simulink model "qpsk_modulation_and_demodulation_1"  (R2024a)
settings: Solver=VariableStepAuto  StartTime=0.0  StopTime=inf  RelTol=1e-3
libraries: simulink x4, dspfdesign x3, dspsigops x3, commsync2 x2, commrflib2 x2, dspxfrm3 x1, commdigbbndpm3 x1, sdrrlib x1, commfilt2 x1, matrix_library x1
settings Model: SimulationMode=accelerator  Creator=digital  LastModifiedBy=opr

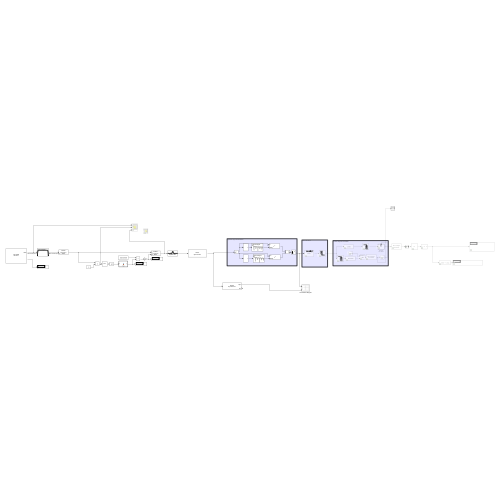
[thumbnail: Simulink's stored preview of the top-level diagram]
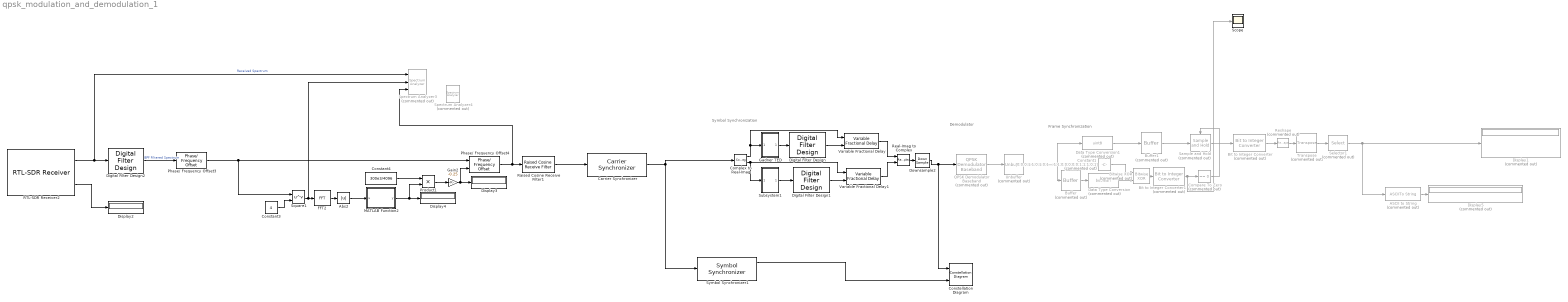
== system qpsk_modulation_and_demodulation_1 ==
  note: Frame Synchronization
  note: Demodulator
  note: Symbol Synchronization
  ASCII to String : ASCIIToString  Commented=on
  Abs2 : Abs  SaturateOnIntegerOverflow=off
  Bit to Integer Converter : simulink/Logic and Bit Operations/Bit to Integer Converter  Commented=on  nbits=8  bitOrder=MSB first  signedOutputValues=Unsigned  outDtype=Inherit via internal rule  outDtypeSigned=Inherit via internal rule
  Bit to Integer Converter1 : simulink/Logic and Bit Operations/Bit to Integer Converter  Commented=on  nbits=32  bitOrder=MSB first  signedOutputValues=Unsigned  outDtype=Inherit via internal rule  outDtypeSigned=Inherit via internal rule
  Bitwise XOR : simulink/Logic and Bit Operations/Bitwise Operator  Commented=on  logicop=XOR  UseBitMask=off  NumInputPorts=2  BitMask=bin2dec('11011001')  BitMaskRealWorld=Stored Integer
      settings: LibrarySourceBlock=|
      | simulink/Quick Insert/Logic and Bit
      | Operations/Bitwise XOR
  Buffer : Buffer  Commented=on  N=32  V=31  OutputFrames=off
  Buffer1 : Buffer  Commented=on  N=160  V=159  OutputFrames=off
  Carrier Synchronizer : commsync2/Carrier Synchronizer  Modulation=QPSK  ModulationPhaseOffset=Auto  CustomPhaseOffset=0  SamplesPerSymbol=2  DampingFactor=0.707  NormalizedLoopBandwidth=0.01  EstimatedPhaseErrorOutputPort=off  SimulateUsing=Code generation
  Compare To Zero : simulink/Logic and Bit Operations/Compare To Zero  Commented=on  relop===  OutDataTypeStr=boolean
  Complex to Real-Imag : ComplexToRealImag
  Constant1 : Constant  Commented=on  Value=[0;0;0;1;1;0;1;0;1;1;0;0;1;1;1;1;1;1;1;1;1;1;0;0;0;0;0;1;1;1;0;1]  VectorParams1D=off  OutDataTypeStr=boolean  SampleTime=1/10e6
  Constant3 : Constant  Value=4
  Constant4 : Constant  Value=300e3/4096
  Constellation Diagram : ConstellationDiagram  NumInputPorts=2  WindowPosition=[1.000000,49.000000,2048.000000,1080.000000,]  ScopeFrameLocation=window  ReferenceConstellation="{[0.7071+0.7071i          -0.7071+0.7071i          -0.7071-0.7071i            0.707-0.7071i][0.7071+0.7071i          -0.7071+0.7071i          -0.7071-0.7071i            0.707-0.7071i]}"  ShowLegend=on
  Data Type Conversion : DataTypeConversion  Commented=on  OutDataTypeStr=boolean  SaturateOnIntegerOverflow=off  RndMeth=Floor
  Data Type Conversion1 : DataTypeConversion  Commented=on  OutDataTypeStr=uint8  SaturateOnIntegerOverflow=off  RndMeth=Floor
  Digital Filter Design : dspfdesign/Digital Filter Design  mwdsp_browser_bugfix_var=off
  Digital Filter Design1 : dspfdesign/Digital Filter Design  mwdsp_browser_bugfix_var=off
  Digital Filter Design2 : dspfdesign/Digital Filter Design  mwdsp_browser_bugfix_var=off
  Display1 : Display  Commented=on
      settings: Format=hex (Stored Integer)
  Display2 : Display
  Display3 : Display
  Display4 : Display
  Display5 : Display  Commented=on
  Downsample2 : DownSample  RateOptions=Allow multirate processing  AllowArbitraryFixedInput=on
  FFT2 : dspxfrm3/FFT  FFTImplementation=Auto  CompMethod=Table lookup  TableOpt=NEW  TableOptActive=Speed  BitRevOrder=off  Normalize=off  InheritFFTLength=on  FFTLength=64  WrapInput=on  roundingMode=Ceiling  overflowMode=off  firstCoeffDataTypeStr=Inherit: Same word length as input  firstCoeffLastDataTypeStr=Inherit: Same word length as input  outputMin=[]  outputMax=[]
  Gadner TED : Subsystem
  Gain2 : Gain  Gain=-0.25
  MATLAB Function2 : MATLAB Function  TreatAsAtomicUnit=on
  Phase/ Frequency Offset3 : commrflib2/Phase// Frequency Offset  phaseOffset=0  freqPort=off  freqOffset=-(300e3)/8
  Phase/ Frequency Offset4 : commrflib2/Phase// Frequency Offset  phaseOffset=0  freqPort=on  freqOffset=500e6
  Product1 : Product
  QPSK Demodulator Baseband : commdigbbndpm3/QPSK Demodulator Baseband  Commented=on  OutType=Bit  DecType=Hard decision  VarSource=Dialog  Variance=1  Dec=Gray  Ph=pi/4  outDtype1=double  outDtype2=uint8  derotateFactorWordLen=16  derotateFactorDataTypeStr=Inherit: Same word length as input  derotateFactorLastDataTypeStr=Inherit: Same word length as input
  RTL-SDR Receiver2 : sdrrlib/RTL-SDR Receiver  IPAddress=0  CenterFrequencySource=Dialog  CenterFrequency=450e6 - (300e3)/4  GainSource=Dialog  Gain=10  ADCRate=300e3  FrequencyCorrection=0  LostSamplesOutputPort=on  LatencyOutputPort=off  OutputDataType=double  FrameLength=4096  EnableBurstMode=off  NumFramesInBurst=50  sobjType=sdrr.internal.SDRRTLReceiverSL  dataUDPPort=-1  ctrlUDPPort=-1  subDeviceList=nosubdev  sdrBlockType=SDRBlockTypeSLT.SDRRxBlock  requester=UNUSED_BY_SFCN  sdrExecutionMode=SDRExecutionModeSLT.ExecModeHW  BypassUserLogic=off  DecimatorSelect=DDC decimator  SourceSelect=RF data  SineAmplitude=16000  EnableInternalClock=off  BypassIQBalance=off  IFBandwidth=40e6  ADCRateSource=Dialog  IntermediateFrequency=0  DecimationFactorSource=Dialog  DecimationFactor=512  RFFrequencyIsTunable=logical(0)  SampleTime=(4096)/(300e3)  IFBandwidthSource=Dialog  SineFrequency=30000  BypassDCBlockingFilter=off  IntermediateFrequencySource=Dialog  IQBalanceCoefficients=64  SkipAllHardwareResetAndInitialization=off  EnableIQCalibrationTable=on  CacheIQCalibrationTable=off  EnableOffsetTuning=off  EnableRTLAGC=off  EnableTestMode=off  EnableTunerAGC=off  FrequencyCorrectionSource=Dialog  NumMLBuffers=128  NumUSBBuffers=16  RTLCrystalFrequency=28800000  TunerCrystalFrequency=28800000
  Raised Cosine Receive Filter1 : commfilt2/Raised Cosine Receive Filter  filtType=Square root  R=0.2  filtSpan=10  N=12  downFactor=6  downOffset=0  filterGain=1  InputProcessing=Columns as channels (frame based)  RateOptions=Allow multirate processing  framing=Mute  checkCoeff=off  variableName=rcRxFilt1  currentFiltSpan=10  D=5  inputOffset=0  sampMode=Mute  saveAsFlag=0  rateMode=Downsampling  checkGain=Normalized  launchFVT=on  roundingMode=Floor  overflowMode=off  coeffDataTypeStr=Inherit: Same word length as input  coeffMin=[]  coeffMax=[]  coeffLastDataTypeStr=Inherit: Same word length as input  accumDataTypeStr=Inherit: Same as product output  accumLastDataTypeStr=Inherit: Same as product output  outputDataTypeStr=Inherit: Same as accumulator  outputMin=[]  outputMax=[]  outputLastDataTypeStr=Inherit: Same as accumulator
  Real-Imag to Complex : RealImagToComplex
  Reshape : Reshape  Commented=on  OutputDimensionality=Row vector (2-D)  OutputDimensions=[1,]
  Sample and Hold : dspsigops/Sample and Hold  Commented=on  trig=Rising edge  initCond=0  latchinput=off
  Scope : Scope
  Selector1 : Selector  Commented=on  InputPortWidth=20  IndexOptions=Index vector (dialog)  Indices=[5:15]  OutputSizes=1
  Spectrum Analyzer3 : SpectrumAnalyzer  Commented=on  NumInputPorts=3  WindowPosition=[111.000000,294.000000,842.000000,726.000000,]  ScopeFrameLocation=window  YLimits=[-283.1209233885463,30.99910976663294]  ShowLegend=on  ExpandToolstrip=on  SelectedToolstripTab=spectrumAnalyzerToolstrip.measurementsTab
  Spectrum Analyzer4 : SpectrumAnalyzer  Commented=on  NumInputPorts=2  WindowPosition=[1367.000000,49.000000,680.000000,1072.000000,]  ScopeFrameLocation=window  YLimits=[-671.6431784277555,755.4983202728769]  ShowLegend=on  SelectedToolstripTab=spectrumAnalyzerToolstrip.measurementsTab
  Square1 : Math  Operator=pow
  Subsystem1 : Subsystem
  Symbol Synchronizer1 : commsync2/Symbol Synchronizer  Modulation=PAM/PSK/QAM  TimingErrorDetector=Gardner (non-data-aided)  SamplesPerSymbol=2  DampingFactor=1  NormalizedLoopBandwidth=0.01  DetectorGain=2.7  TimingErrorOutputPort=on  SimulateUsing=Interpreted execution
  Transpose : matrix_library/Transpose  Commented=on
  Unbuffer : Unbuffer  Commented=on
  Variable Fractional Delay : dspsigops/Variable Fractional Delay  mode=OBSOLETE  modeActive=Linear  L=4  FarrowL=4  R=10  alpha=1  dmax=100  InputProcessing=Columns as channels (frame based)  ic=0  noDFT=off  fallbackFIR=Clip to the minimum value necessary for centered kernel  fallbackFarrow=Clip to the minimum value necessary for centered kernel  roundingMode=Zero  overflowMode=off
  Variable Fractional Delay1 : dspsigops/Variable Fractional Delay  mode=OBSOLETE  modeActive=Linear  L=4  FarrowL=4  R=10  alpha=1  dmax=100  InputProcessing=Columns as channels (frame based)  ic=0  noDFT=off  fallbackFIR=Clip to the minimum value necessary for centered kernel  fallbackFarrow=Clip to the minimum value necessary for centered kernel  roundingMode=Zero  overflowMode=off
  wires:
  Complex to Real-Imag/1 -> Gadner TED/1(In1), Variable Fractional Delay/1
  Complex to Real-Imag/2 -> Variable Fractional Delay1/1, Subsystem1/1(In1)
  Subsystem1/1(Out1) -> Digital Filter Design1/1
  Gadner TED/1(Out1) -> Digital Filter Design/1
  Digital Filter Design/1 -> Variable Fractional Delay/2
  Digital Filter Design1/1 -> Variable Fractional Delay1/2
  Bitwise XOR/1 -> Bit to Integer Converter1/1
  QPSK Demodulator Baseband/1 -> Unbuffer/1
  Unbuffer/1 -> Buffer/1, Data Type Conversion1/1
  Buffer/1 -> Data Type Conversion/1
  Variable Fractional Delay/1 -> Real-Imag to Complex/1
  Variable Fractional Delay1/1 -> Real-Imag to Complex/2
  Real-Imag to Complex/1 -> Downsample2/1
  Downsample2/1 -> Constellation Diagram/1, QPSK Demodulator Baseband/1
  Data Type Conversion/1 -> Bitwise XOR/2
  Constant1/1 -> Bitwise XOR/1
  Buffer1/1 -> Sample and Hold/1
  Data Type Conversion1/1 -> Buffer1/1
  Sample and Hold/1 -> Bit to Integer Converter/1
  Reshape/1 -> Transpose/1
  Bit to Integer Converter/1 -> Reshape/1
  Transpose/1 -> Selector1/1
  MATLAB Function2/1(y) -> Display4/1, Product1/2
  RTL-SDR Receiver2/2 -> Display2/1
  Phase/ Frequency Offset4/1 -> Spectrum Analyzer3/3, Raised Cosine Receive Filter1/1
  Product1/1 -> Gain2/1
  Abs2/1 -> MATLAB Function2/1(u)
  RTL-SDR Receiver2/1 -> Spectrum Analyzer3/1, Digital Filter Design2/1  "Received Spectrum"
  FFT2/1 -> Abs2/1
  Constant3/1 -> Square1/2
  Constant4/1 -> Product1/1
  Gain2/1 -> Display3/1, Phase/ Frequency Offset4/2
  Square1/1 -> Spectrum Analyzer3/2, FFT2/1
  Phase/ Frequency Offset3/1 -> Square1/1, Phase/ Frequency Offset4/1
  Digital Filter Design2/1 -> Phase/ Frequency Offset3/1  "BPF Filtered Spectrum"
  Raised Cosine Receive Filter1/1 -> Carrier Synchronizer/1
  Compare To Zero/1 -> Sample and Hold/Trigger
  Bit to Integer Converter1/1 -> Scope/1, Compare To Zero/1
  ASCII to String/1 -> Display5/1
  Selector1/1 -> ASCII to String/1, Display1/1
  Carrier Synchronizer/1 -> Symbol Synchronizer1/1, Complex to Real-Imag/1
  Symbol Synchronizer1/1 -> Constellation Diagram/2

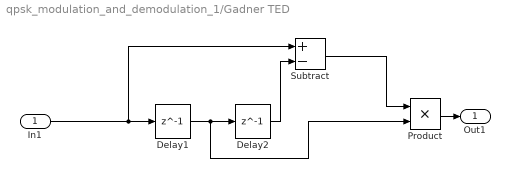
== system qpsk_modulation_and_demodulation_1/Gadner TED ==
  In1 : Inport
  Delay1 : Delay  DelayLength=1  InitialCondition=0
  Delay2 : Delay  DelayLength=1  InitialCondition=0
  Product : Product
  Subtract : Sum  Inputs=+-
  Out1 : Outport
  wires:
  Product/1 -> Out1/1
  Delay1/1 -> Product/2, Delay2/1
  In1/1 -> Subtract/1, Delay1/1
  Subtract/1 -> Product/1
  Delay2/1 -> Subtract/2

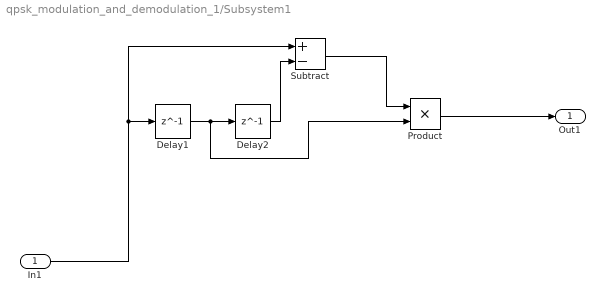
== system qpsk_modulation_and_demodulation_1/Subsystem1 ==
  In1 : Inport
  Delay1 : Delay  DelayLength=1  InitialCondition=0
  Delay2 : Delay  DelayLength=1  InitialCondition=0
  Product : Product
  Subtract : Sum  Inputs=+-
  Out1 : Outport
  wires:
  Delay2/1 -> Subtract/2
  Subtract/1 -> Product/1
  In1/1 -> Delay1/1, Subtract/1
  Delay1/1 -> Delay2/1, Product/2
  Product/1 -> Out1/1

== matlab function qpsk_modulation_and_demodulation_1/MATLAB Function2 ==
  data: u input; y output
function y = fcn(u)

[M,idx] = max(u);
if idx > 2048
    y = 4096-idx;
else
    y=idx;
end
